simulink model "Test_Sequence_Block_Example"  (R2025b)
settings: Solver=VariableStepAuto  StartTime=0.0  StopTime=10.0  RelTol=1e-3
settings Model: Creator=P28500  LastModifiedBy=P28500

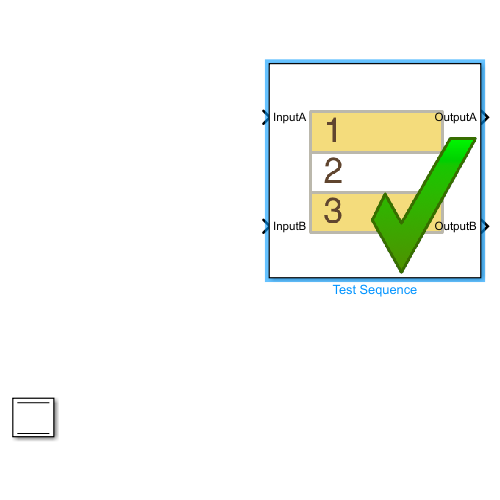
[thumbnail: Simulink's stored preview of the top-level diagram]
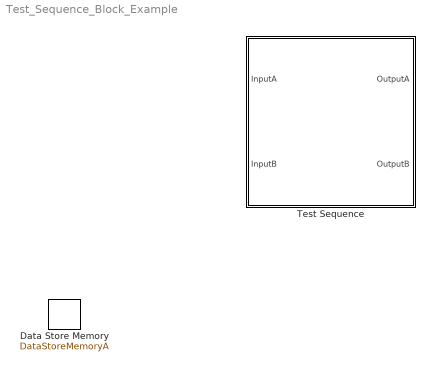
== system Test_Sequence_Block_Example ==
  Data Store Memory : DataStoreMemory  DataStoreName=DataStoreMemoryA  WriteAfterWriteMsg=warning  ShowAdditionalParam=off  OutDataTypeStr=double
  Test Sequence : Test Sequence  TreatAsAtomicUnit=on

== stateflow chart Test_Sequence_Block_Example/Test Sequence ==
  state step_1
    OutputA = t
    OutputB = 6
  state step_2
    OutputA = t
    OutputB= 3
  state step_3
    OutputA = t
    OutputB = 7
  (default) -> step_1
  (junction 48) -> step_1
  (junction 54) -> (junction 48)
  step_1 -> step_2 : [
      | InputA == 0
      | ]
  step_2 -> step_3 : [
      | InputA == 1
      | ]
  step_3 -> (junction 54) : [
      | InputA == 2
      | ]
  data: OutputA output double; OutputB output double; InputA input double; InputB input double; LocalA local double =0; ConstantA constant double =1; ParameterA parameter double
